simulink model "iver_model"  (R2016b)
settings: Solver=VariableStepAuto  StartTime=0.0  StopTime=10.0  RelTol=1e-3
values from neighbouring files (symbols this model uses):
  Ix = 0.05    [belugaSimulation.m]    (also in belugaStep.m; iverSimulation.m = 0; matlab.mat)
  Iy = 2.05    [belugaSimulation.m]    (also in belugaStep.m; iverSimulation.m = 0; matlab.mat)
  Iz = 2.06    [belugaSimulation.m]    (also in belugaStep.m; iverSimulation.m = 0; matlab.mat)
  K_pdot = -0.0704    [belugaSimulation.m]    (also in belugaStep.m; iverSimulation.m = 0; matlab.mat)
  m = 16.7/2.2    (= 7.59090909091)    [belugaSimulation.m]    (also in belugaStep.m = 4.2173; gps_state_est.m = 1; iverSimulation.m = 0; lin_test.m = 20.2)
  M_qdot = -3.2455    [belugaSimulation.m]    (also in belugaStep.m; iverSimulation.m = 0; matlab.mat)
  M_wdot = 2.5656    [belugaSimulation.m]    (also in belugaStep.m; iverSimulation.m = 0; matlab.mat)
  N_rdot = -3.2455    [belugaSimulation.m]    (also in belugaStep.m; iverSimulation.m = 0; matlab.mat)
  N_vdot = -2.5656    [belugaSimulation.m]    (also in belugaStep.m; iverSimulation.m = 0; matlab.mat)
  X_udot = -0.51334    [belugaSimulation.m]    (also in belugaStep.m; iverSimulation.m = 0; matlab.mat)
  xg = 0    [belugaSimulation.m]    (also in belugaStep.m; iverSimulation.m; matlab.mat)
  Y_rdot = -2.5656    [belugaSimulation.m]    (also in belugaStep.m; iverSimulation.m = 0; matlab.mat)
  Y_vdot = -23.8314    [belugaSimulation.m]    (also in belugaStep.m; iverSimulation.m = 0; matlab.mat)
  Z_qdot = 2.5656    [belugaSimulation.m]    (also in belugaStep.m; iverSimulation.m = 0; matlab.mat)
  Z_wdot = -23.8314    [belugaSimulation.m]    (also in belugaStep.m; iverSimulation.m = 0; matlab.mat)
  zg = 0    [belugaSimulation.m]    (also in belugaStep.m; iverSimulation.m; matlab.mat)
libraries: dspinverses x1
settings Model: Creator=HMCLoaner  LastModifiedBy=HMCLoaner

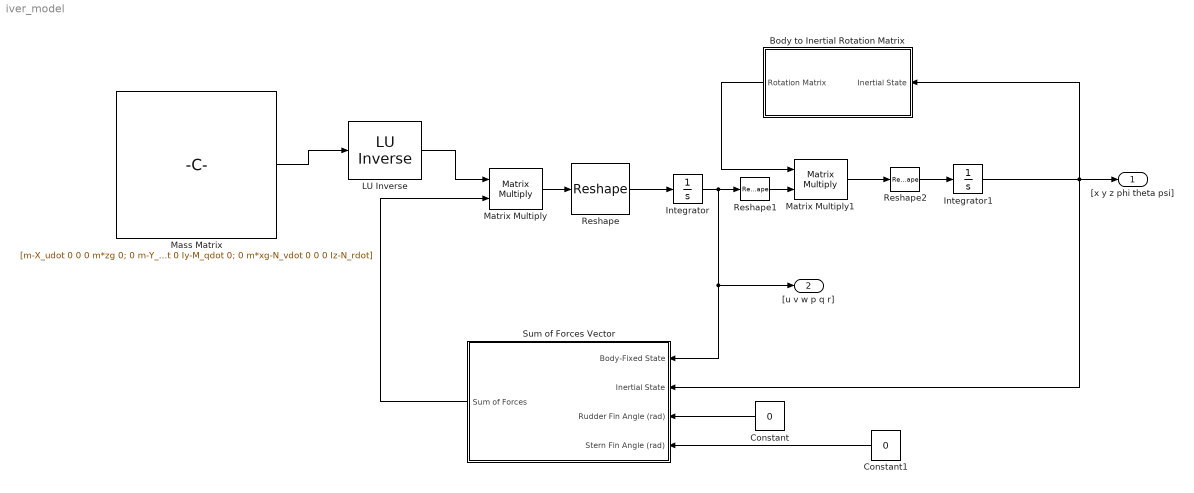
== system iver_model ==
  " LU Inverse" : dspinverses/ LU Inverse
  Body to Inertial Rotation Matrix : Subsystem
  Constant : Constant  Value=0
  Constant1 : Constant  Value=0
  Integrator : Integrator  InitialCondition=[0 0 0 0 0 0]'
  Integrator1 : Integrator  InitialCondition=[0 0 0 0 0 0]'
  "Mass Matrix " : Constant  Value=[m-X_udot 0 0 0 m*zg 0; 0 m-Y_vdot 0 -m*zg 0 m*xg-Y_rdot; 0 0 m-Z_wdot 0 -m*xg-Z_qdot 0; 0 -m*zg 0 Ix-K_pdot 0 0; m*zg 0 -m*xg-M_wdot 0 Iy-M_qdot 0; 0 m*xg-N_vdot 0 0 0 Iz-N_rdot]  VectorParams1D=off
  Matrix Multiply : Product  Multiplication=Matrix(*)
  Matrix Multiply1 : Product  Multiplication=Matrix(*)
  Reshape : Reshape  OutputDimensions=3
  Reshape1 : Reshape  OutputDimensions=[1,6]
  Reshape2 : Reshape  OutputDimensions=[6,1]
  Sum of Forces Vector : Subsystem
  "[x y z phi theta psi]" : Outport
  "[u v w p q r]" : Outport  Port=2
  wires:
  Reshape/1 -> Integrator/1
  Matrix Multiply/1 -> Reshape/1
  " LU Inverse"/1 -> Matrix Multiply/1
  Integrator/1 -> Sum of Forces Vector/1(Body-Fixed State), "[u v w p q r]"/1, Reshape1/1
  Reshape1/1 -> Matrix Multiply1/2
  Reshape2/1 -> Integrator1/1
  Matrix Multiply1/1 -> Reshape2/1
  "Mass Matrix "/1 -> " LU Inverse"/1
  Body to Inertial Rotation Matrix/1(Rotation Matrix) -> Matrix Multiply1/1
  Sum of Forces Vector/1(Sum of Forces) -> Matrix Multiply/2
  Constant/1 -> Sum of Forces Vector/3(Rudder Fin Angle (rad))
  Constant1/1 -> Sum of Forces Vector/4(Stern Fin Angle (rad))
  Integrator1/1 -> Sum of Forces Vector/2(Inertial State), Body to Inertial Rotation Matrix/1(Inertial State), "[x y z phi theta psi]"/1

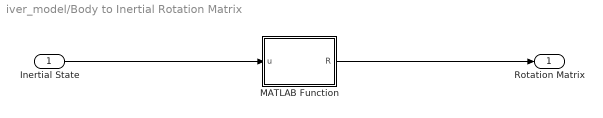
== system iver_model/Body to Inertial Rotation Matrix ==
  Inertial State : Inport
  MATLAB Function : MATLAB Function  TreatAsAtomicUnit=on
  Rotation Matrix : Outport  PortDimensions=[6,6]
  wires:
  MATLAB Function/1(R) -> Rotation Matrix/1
  Inertial State/1 -> MATLAB Function/1(u)

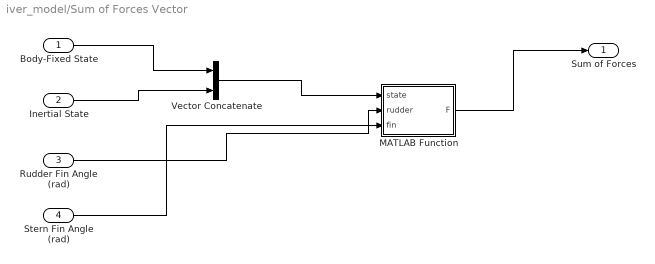
== system iver_model/Sum of Forces Vector ==
  Body-Fixed State : Inport
  Inertial State : Inport  Port=2
  Rudder Fin Angle (rad) : Inport  Port=3
  Stern Fin Angle (rad) : Inport  Port=4
  MATLAB Function : MATLAB Function  TreatAsAtomicUnit=on
  Vector Concatenate : Concatenate
  Sum of Forces : Outport
  wires:
  Body-Fixed State/1 -> Vector Concatenate/1
  Inertial State/1 -> Vector Concatenate/2
  Vector Concatenate/1 -> MATLAB Function/1(state)
  Rudder Fin Angle (rad)/1 -> MATLAB Function/2(rudder)
  Stern Fin Angle (rad)/1 -> MATLAB Function/3(fin)
  MATLAB Function/1(F) -> Sum of Forces/1

== matlab function iver_model/Sum of Forces Vector/MATLAB Function ==
  data: state input; F output; rudder input; fin input
function F = fcn(state, rudder, fin)
    
    %% Constants
    % Vehicle measure parameters
    W = 183.845;
    B = 185.8;
    m = W/9.8;
    X_prop = 65; % constant input thrust
    K_prop = 0; %TODO moment of prop
    
    %Measured or Estimated Centers of Buoyancy and Gravity
    xcg = 0;
    ycg = 0;
    zcg = 0.0022606;
    xcb = -0.602488;
    ycb = 0;
    zcb = 0.000762;
    
    %Fin characteristic parameters:
    i2m = 0.0254; 
    rho = 1.03*10^(3); %seawater density (kg/m^3)
    fin1 = 2.54*i2m;
    fin2 = 1.92*i2m;
    fin3 = 5.7*i2m;
    fin4 = 1.26*i2m;
    fin5 = 3.51*i2m;
    fin6 = 4.5*i2m;
        
    %****Iver2 Values*****    
    a = 8*i2m;
    a_offset = 0*i2m;
    b = 33.375*i2m;
    c = 7.34*i2m;
    c_offset = 1.04*i2m;
    d = 5.83*i2m;
    xn = abs(xcb)-(a-a_offset);
    xt2 = -(b-xn);
    xt = xt2 - (c - c_offset);
    xf2 = xt+fin6;
    %*********************
    Sfin = 1/2*(fin1-fin2)*(fin6-fin4)+1/2*(fin6-fin5)*(fin3-fin1)+...
     (  fin6-fin4)*(fin3-fin1); %control fin planform area
    xfin = xf2; %fin moment arm wrt origin at COB
    
    %Define Fin Lift coefficients
    SpanAve = 1/2*( (fin3-fin2)+(fin3-fin1) ); %avg span of one fin
    ARe = 2*(SpanAve^2)/Sfin; %Effective wing aspect ratio
    Cla = inv( 1/(2*0.9*pi) + 1/(pi*ARe) );
    Yuvf = -1/2*rho*Cla*Sfin; %kg/m
    Y_uudr = -Yuvf; %kg/(m*rad)
    Zuwf = -1/2*rho*Cla*Sfin; %kg/m
    Z_uuds = Zuwf; %kg/(m*rad)
    Zuqf = 1/2*rho*Cla*Sfin*xfin; %kg/rad
    Yurf = -Zuqf; %kg/rad
    Muwf = 1/2*rho*Cla*Sfin*xfin; %kg
    M_uuds = Muwf; %kg/rad
    Nuvf = -1/2*rho*Cla*Sfin*xfin; %kg
    N_uudr = -Nuvf; %kg/rad
    Nurf = -1/2*rho*Cla*Sfin*xfin^2;%kg*m/rad
    Muqf = Nurf; %kg*m/rad
    
    
    % defining states
    u = state(1);
    v = state(2);
    w = state(3);
    p = state(4);
    q = state(5);
    r = state(6);
    
    x = state(7);
    y = state(8);
    z = state(9);
    phi = state(10);
    theta = state(11);
    psi = state(12);
    
    % Hydrostatic forces
    X_hs = -(W-B)*sin(theta);
    Y_hs = (W-B)*sin(phi)*cos(theta);
    Z_hs = (W-B)*cos(phi)*cos(theta);
    K_hs = (ycg*W-ycb*B)*cos(theta)*cos(phi)-(zcg*W-zcb*B)*cos(theta)*sin(phi);
    M_hs = -(xcg*W-xcb*B)*cos(theta)*cos(phi)-(zcg*W-zcb*B)*sin(theta);
    N_hs = (xcg*W-xcb*B)*cos(theta)*sin(phi)-(ycg*W-ycb*B)*sin(theta);
    
    % Control Forces
    X_c = X_prop;
    Y_c = Y_uudr*u^2*rudder;
    Z_c = Z_uuds*u^2*fin;
    K_c = K_prop;
    M_c = M_uuds*u^2*fin;
    N_c = N_uudr*u^2*rudder;
    
    % output force vector
    X = X_hs+X_c;
    Y = Y_hs+Y_c;
    Z = Z_hs+Z_c;
    K = K_hs+K_c;
    M = M_hs+M_c;
    N = N_hs+N_c;
    F = [X Y Z K M N]'; 
    F = [1 0 0 0 0 0]';
end

== matlab function iver_model/Body to Inertial Rotation Matrix/MATLAB Function ==
  data: u input; R output
function R = fcn(u)
    % Inputs
    x = u(1);
    y = u(2);
    z = u(3);
    phi = u(4);
    theta = u(5);
    psi = u(6);
    
    % transformation
    cosphi = cos(phi);
    sinphi = sin(phi);
    costheta = cos(theta);
    sintheta = sin(theta);
    cospsi = cos(psi);
    sinpsi = sin(psi);

    R = zeros(6,6);
    R(1,1) = cospsi.*cosphi-costheta.*sinphi.*sinpsi;
    R(1,2) = sinphi.*cospsi+costheta.*cosphi.*sinpsi;
    R(1,3) = sintheta.*sinpsi;

    R(2,1) = -cosphi.*sinpsi-costheta.*cospsi.*sinphi;
    R(2,2) = -sinpsi.*sinphi+costheta.*cosphi.*cospsi;
    R(2,3) = sintheta.*cospsi;

    R(3,1) = sinphi.*sintheta;
    R(3,2) = -cosphi.*sintheta;
    R(3,3) = costheta;
    
    R(4,4) = 1;
    R(5,5) = 1;
    R(6,6) = 1;
end
